simulink model "ROPOD_4Wheel_Tdistkinb_cntr_vel_filter_test"  (R2017b)
settings: Solver=FixedStepAuto  StartTime=0.0  StopTime=Inf  FixedStep=Ts  RelTol=1e-3
PreLoadFcn:
  | init_model
InitFcn:
  | init_model
values from neighbouring files (symbols this model uses):
  FFtheta_intia = 0    [init_model.m]
  FFxy_mass = 0*80    (= 0)    [init_model.m]
  max_hw_tau = 7.0    (= 7)    [init_model.m]
  max_ropod_sw_force = 500    [init_model.m]
  max_ropod_sw_tau = 250    [init_model.m]
  Nwheels = 4    [Jqwl_numeric_function.m]    (also in S_matrix.m; extract_kinmodel_parameters.m; init_model.m; tau_optimal_dist_vec_fun.m)
  pivot_offs_sws = [3.835 3.465 2.059 0.357]    [init_model.m]
  SW_COM1_ENABLE1 = hex2dec('0001')    [init_model.m]
  SW_COM1_ENABLE2 = hex2dec('0002')    [init_model.m]
  SW_COM1_MODE_TORQUE = bitshift(hex2dec('0000'),2)    [init_model.m]
  SW_COM1_MODE_VELOCITY = bitshift(hex2dec('0002'),2)    [init_model.m]
  SW_COM1_USE_TS = hex2dec('8000')    [init_model.m]
  sw_tau_2_curr = 1/motor_physical_parameters.torqueconstant.value    [init_model.m]
  Taucompfactor = 2.0    (= 2)    [init_model.m]
  Tinit = 5    [init_model.m]
  Ts = 0.001    [init_model.m]
  Tsp = 1    [init_model.m]
undefined symbols (not defined in the file or in its folder): DiscIntNeverNeededParam, Pose, ropod_kinmodel_param, Twist
libraries: robotlib x48, simulink x46, cstblocks x23, dspsigops x12, SOEM_EtherCAT_Lib x5, robotcorelib x1
(part 4 of 4)

== system ROPOD_4Wheel_Tdistkinb_cntr_vel_filter_test/Non-ROS Ropod Controller/wheel vel cntr/Wheels Velocity controller/G_I_LL_LPF Controller3/Shapeit Lead-Lag (Tustin) ==
  In : Inport
  fz : Inport  Port=2
  fp : Inport  Port=3
  Add : Sum  Inputs=+-
  Constant1 : Constant
  Constant2 : Constant  Value=0
  Constant4 : Constant
  Divide : Product  Inputs=*/
  Divide1 : Product  Inputs=/*
  Gain1 : Gain  Gain=2*pi
  Gain2 : Gain  Gain=2*pi
  PID Controller3 : simulink/Continuous/PID Controller  Controller=PID  TimeDomain=Discrete-time  SampleTime=Ts  IntegratorMethod=Trapezoidal  FilterMethod=Trapezoidal  Form=Parallel  UseFilter=on  ControllerParametersSource=external  P=0.4  I=0.4*2*pi*3  D=0  N=100  InitialConditionSource=internal  InitialConditionForIntegrator=0  InitialConditionForFilter=0  ExternalReset=none  LimitOutput=off  UpperSaturationLimit=max_hw_tau  LowerSaturationLimit=-max_hw_tau  LinearizeAsGain=on  AntiWindupMode=clamping  Kb=1  TrackingMode=off  Kt=1  PParamMin=[]  PParamMax=[]  IParamMin=[]  IParamMax=[]  DParamMin=[]  DParamMax=[]  NParamMin=[]  NParamMax=[]  KbParamMin=[]  KbParamMax=[]  KtParamMin=[]  KtParamMax=[]  POutMin=[]  POutMax=[]  IOutMin=[]  IOutMax=[]  DOutMin=[]  DOutMax=[]  NOutMin=[]  NOutMax=[]  KbOutMin=[]  KbOutMax=[]  KtOutMin=[]  KtOutMax=[]  IntegratorOutMin=[]  IntegratorOutMax=[]  FilterOutMin=[]  FilterOutMax=[]  SumOutMin=[]  SumOutMax=[]  SumI1OutMin=[]  SumI1OutMax=[]  SumI2OutMin=[]  SumI2OutMax=[]  SumI3OutMin=[]  SumI3OutMax=[]  SumDOutMin=[]  SumDOutMax=[]  SaturationOutMin=[]  SaturationOutMax=[]  IntegratorContinuousStateAttributes=''  IntegratorStateMustResolveToSignalObject=off  IntegratorRTWStateStorageClass=Auto  FilterContinuousStateAttributes=''  FilterStateMustResolveToSignalObject=off  FilterRTWStateStorageClass=Auto  DifferentiatorICPrevScaledInput=0  DifferentiatorOutMin=[]  DifferentiatorOutMax=[]  InitialConditionSetting=State (most efficient)  FilterDiffOutCoefMin=[]  FilterDiffOutCoefMax=[]  SumDenOutMin=[]  SumDenOutMax=[]  SumNumOutMin=[]  SumNumOutMax=[]  ReciprocalOutMin=[]  ReciprocalOutMax=[]  DivideOutMin=[]  DivideOutMax=[]  TunerSelectOption=Transfer Function Based (PID Tuner App)
  Out : Outport
  wires:
  Divide1/1 -> PID Controller3/4
  Add/1 -> Divide1/2
  Constant1/1 -> Add/1
  Divide/1 -> Add/2
  Gain2/1 -> Divide/1, Divide1/1
  Constant2/1 -> PID Controller3/3
  Gain1/1 -> Divide/2, PID Controller3/5
  fp/1 -> Gain1/1
  fz/1 -> Gain2/1
  PID Controller3/1 -> Out/1
  In/1 -> PID Controller3/1
  Constant4/1 -> PID Controller3/2

== system ROPOD_4Wheel_Tdistkinb_cntr_vel_filter_test/Non-ROS Ropod Controller/wheel vel cntr/Wheels Velocity controller/G_I_LL_LPF Controller4/Shapeit Integrator (Tustin) ==
  In : Inport
  I_fhz : Inport  Port=2
  reset : Inport  Port=3
  Constant : Constant  Value=0
  Constant4 : Constant
  Constant5 : Constant  Value=0
  Gain2 : Gain  Gain=2*pi
  PID Controller3 : simulink/Continuous/PID Controller  Controller=PID  TimeDomain=Discrete-time  SampleTime=Ts  IntegratorMethod=Trapezoidal  FilterMethod=Trapezoidal  Form=Parallel  UseFilter=on  ControllerParametersSource=external  P=0.4  I=0.4*2*pi*3  D=0  N=100  InitialConditionSource=internal  InitialConditionForIntegrator=0  InitialConditionForFilter=0  ExternalReset=level  LimitOutput=on  UpperSaturationLimit=max_hw_tau  LowerSaturationLimit=-max_hw_tau  LinearizeAsGain=on  AntiWindupMode=clamping  Kb=1  TrackingMode=off  Kt=1  PParamMin=[]  PParamMax=[]  IParamMin=[]  IParamMax=[]  DParamMin=[]  DParamMax=[]  NParamMin=[]  NParamMax=[]  KbParamMin=[]  KbParamMax=[]  KtParamMin=[]  KtParamMax=[]  POutMin=[]  POutMax=[]  IOutMin=[]  IOutMax=[]  DOutMin=[]  DOutMax=[]  NOutMin=[]  NOutMax=[]  KbOutMin=[]  KbOutMax=[]  KtOutMin=[]  KtOutMax=[]  IntegratorOutMin=[]  IntegratorOutMax=[]  FilterOutMin=[]  FilterOutMax=[]  SumOutMin=[]  SumOutMax=[]  SumI1OutMin=[]  SumI1OutMax=[]  SumI2OutMin=[]  SumI2OutMax=[]  SumI3OutMin=[]  SumI3OutMax=[]  SumDOutMin=[]  SumDOutMax=[]  SaturationOutMin=[]  SaturationOutMax=[]  IntegratorContinuousStateAttributes=''  IntegratorStateMustResolveToSignalObject=off  IntegratorRTWStateStorageClass=Auto  FilterContinuousStateAttributes=''  FilterStateMustResolveToSignalObject=off  FilterRTWStateStorageClass=Auto  DifferentiatorICPrevScaledInput=0  DifferentiatorOutMin=[]  DifferentiatorOutMax=[]  InitialConditionSetting=State (most efficient)  FilterDiffOutCoefMin=[]  FilterDiffOutCoefMax=[]  SumDenOutMin=[]  SumDenOutMax=[]  SumNumOutMin=[]  SumNumOutMax=[]  ReciprocalOutMin=[]  ReciprocalOutMax=[]  DivideOutMin=[]  DivideOutMax=[]  TunerSelectOption=Transfer Function Based (PID Tuner App)
  Product4 : Product
  Out : Outport
  wires:
  I_fhz/1 -> Product4/2
  Product4/1 -> Gain2/1
  reset/1 -> PID Controller3/6
  Gain2/1 -> PID Controller3/3
  PID Controller3/1 -> Out/1
  In/1 -> PID Controller3/1
  Constant4/1 -> Product4/1, PID Controller3/2
  Constant5/1 -> PID Controller3/5
  Constant/1 -> PID Controller3/4

== system ROPOD_4Wheel_Tdistkinb_cntr_vel_filter_test/Non-ROS Ropod Controller/wheel vel cntr/Wheels Velocity controller/G_I_LL_LPF Controller4/Shapeit Lead-Lag (Tustin) ==
  In : Inport
  fz : Inport  Port=2
  fp : Inport  Port=3
  Add : Sum  Inputs=+-
  Constant1 : Constant
  Constant2 : Constant  Value=0
  Constant4 : Constant
  Divide : Product  Inputs=*/
  Divide1 : Product  Inputs=/*
  Gain1 : Gain  Gain=2*pi
  Gain2 : Gain  Gain=2*pi
  PID Controller3 : simulink/Continuous/PID Controller  Controller=PID  TimeDomain=Discrete-time  SampleTime=Ts  IntegratorMethod=Trapezoidal  FilterMethod=Trapezoidal  Form=Parallel  UseFilter=on  ControllerParametersSource=external  P=0.4  I=0.4*2*pi*3  D=0  N=100  InitialConditionSource=internal  InitialConditionForIntegrator=0  InitialConditionForFilter=0  ExternalReset=none  LimitOutput=off  UpperSaturationLimit=max_hw_tau  LowerSaturationLimit=-max_hw_tau  LinearizeAsGain=on  AntiWindupMode=clamping  Kb=1  TrackingMode=off  Kt=1  PParamMin=[]  PParamMax=[]  IParamMin=[]  IParamMax=[]  DParamMin=[]  DParamMax=[]  NParamMin=[]  NParamMax=[]  KbParamMin=[]  KbParamMax=[]  KtParamMin=[]  KtParamMax=[]  POutMin=[]  POutMax=[]  IOutMin=[]  IOutMax=[]  DOutMin=[]  DOutMax=[]  NOutMin=[]  NOutMax=[]  KbOutMin=[]  KbOutMax=[]  KtOutMin=[]  KtOutMax=[]  IntegratorOutMin=[]  IntegratorOutMax=[]  FilterOutMin=[]  FilterOutMax=[]  SumOutMin=[]  SumOutMax=[]  SumI1OutMin=[]  SumI1OutMax=[]  SumI2OutMin=[]  SumI2OutMax=[]  SumI3OutMin=[]  SumI3OutMax=[]  SumDOutMin=[]  SumDOutMax=[]  SaturationOutMin=[]  SaturationOutMax=[]  IntegratorContinuousStateAttributes=''  IntegratorStateMustResolveToSignalObject=off  IntegratorRTWStateStorageClass=Auto  FilterContinuousStateAttributes=''  FilterStateMustResolveToSignalObject=off  FilterRTWStateStorageClass=Auto  DifferentiatorICPrevScaledInput=0  DifferentiatorOutMin=[]  DifferentiatorOutMax=[]  InitialConditionSetting=State (most efficient)  FilterDiffOutCoefMin=[]  FilterDiffOutCoefMax=[]  SumDenOutMin=[]  SumDenOutMax=[]  SumNumOutMin=[]  SumNumOutMax=[]  ReciprocalOutMin=[]  ReciprocalOutMax=[]  DivideOutMin=[]  DivideOutMax=[]  TunerSelectOption=Transfer Function Based (PID Tuner App)
  Out : Outport
  wires:
  Constant4/1 -> PID Controller3/2
  In/1 -> PID Controller3/1
  PID Controller3/1 -> Out/1
  fz/1 -> Gain2/1
  fp/1 -> Gain1/1
  Gain1/1 -> PID Controller3/5, Divide/2
  Constant2/1 -> PID Controller3/3
  Gain2/1 -> Divide1/1, Divide/1
  Divide/1 -> Add/2
  Constant1/1 -> Add/1
  Add/1 -> Divide1/2
  Divide1/1 -> PID Controller3/4

== system ROPOD_4Wheel_Tdistkinb_cntr_vel_filter_test/Non-ROS Ropod Controller/wheel vel cntr/Wheels Velocity controller/G_I_LL_LPF Controller5/Shapeit Integrator (Tustin) ==
  In : Inport
  I_fhz : Inport  Port=2
  reset : Inport  Port=3
  Constant : Constant  Value=0
  Constant4 : Constant
  Constant5 : Constant  Value=0
  Gain2 : Gain  Gain=2*pi
  PID Controller3 : simulink/Continuous/PID Controller  Controller=PID  TimeDomain=Discrete-time  SampleTime=Ts  IntegratorMethod=Trapezoidal  FilterMethod=Trapezoidal  Form=Parallel  UseFilter=on  ControllerParametersSource=external  P=0.4  I=0.4*2*pi*3  D=0  N=100  InitialConditionSource=internal  InitialConditionForIntegrator=0  InitialConditionForFilter=0  ExternalReset=level  LimitOutput=on  UpperSaturationLimit=max_hw_tau  LowerSaturationLimit=-max_hw_tau  LinearizeAsGain=on  AntiWindupMode=clamping  Kb=1  TrackingMode=off  Kt=1  PParamMin=[]  PParamMax=[]  IParamMin=[]  IParamMax=[]  DParamMin=[]  DParamMax=[]  NParamMin=[]  NParamMax=[]  KbParamMin=[]  KbParamMax=[]  KtParamMin=[]  KtParamMax=[]  POutMin=[]  POutMax=[]  IOutMin=[]  IOutMax=[]  DOutMin=[]  DOutMax=[]  NOutMin=[]  NOutMax=[]  KbOutMin=[]  KbOutMax=[]  KtOutMin=[]  KtOutMax=[]  IntegratorOutMin=[]  IntegratorOutMax=[]  FilterOutMin=[]  FilterOutMax=[]  SumOutMin=[]  SumOutMax=[]  SumI1OutMin=[]  SumI1OutMax=[]  SumI2OutMin=[]  SumI2OutMax=[]  SumI3OutMin=[]  SumI3OutMax=[]  SumDOutMin=[]  SumDOutMax=[]  SaturationOutMin=[]  SaturationOutMax=[]  IntegratorContinuousStateAttributes=''  IntegratorStateMustResolveToSignalObject=off  IntegratorRTWStateStorageClass=Auto  FilterContinuousStateAttributes=''  FilterStateMustResolveToSignalObject=off  FilterRTWStateStorageClass=Auto  DifferentiatorICPrevScaledInput=0  DifferentiatorOutMin=[]  DifferentiatorOutMax=[]  InitialConditionSetting=State (most efficient)  FilterDiffOutCoefMin=[]  FilterDiffOutCoefMax=[]  SumDenOutMin=[]  SumDenOutMax=[]  SumNumOutMin=[]  SumNumOutMax=[]  ReciprocalOutMin=[]  ReciprocalOutMax=[]  DivideOutMin=[]  DivideOutMax=[]  TunerSelectOption=Transfer Function Based (PID Tuner App)
  Product4 : Product
  Out : Outport
  wires:
  Constant/1 -> PID Controller3/4
  Constant5/1 -> PID Controller3/5
  Constant4/1 -> PID Controller3/2, Product4/1
  In/1 -> PID Controller3/1
  PID Controller3/1 -> Out/1
  Gain2/1 -> PID Controller3/3
  reset/1 -> PID Controller3/6
  Product4/1 -> Gain2/1
  I_fhz/1 -> Product4/2

== system ROPOD_4Wheel_Tdistkinb_cntr_vel_filter_test/Non-ROS Ropod Controller/wheel vel cntr/Wheels Velocity controller/G_I_LL_LPF Controller5/Shapeit Lead-Lag (Tustin) ==
  In : Inport
  fz : Inport  Port=2
  fp : Inport  Port=3
  Add : Sum  Inputs=+-
  Constant1 : Constant
  Constant2 : Constant  Value=0
  Constant4 : Constant
  Divide : Product  Inputs=*/
  Divide1 : Product  Inputs=/*
  Gain1 : Gain  Gain=2*pi
  Gain2 : Gain  Gain=2*pi
  PID Controller3 : simulink/Continuous/PID Controller  Controller=PID  TimeDomain=Discrete-time  SampleTime=Ts  IntegratorMethod=Trapezoidal  FilterMethod=Trapezoidal  Form=Parallel  UseFilter=on  ControllerParametersSource=external  P=0.4  I=0.4*2*pi*3  D=0  N=100  InitialConditionSource=internal  InitialConditionForIntegrator=0  InitialConditionForFilter=0  ExternalReset=none  LimitOutput=off  UpperSaturationLimit=max_hw_tau  LowerSaturationLimit=-max_hw_tau  LinearizeAsGain=on  AntiWindupMode=clamping  Kb=1  TrackingMode=off  Kt=1  PParamMin=[]  PParamMax=[]  IParamMin=[]  IParamMax=[]  DParamMin=[]  DParamMax=[]  NParamMin=[]  NParamMax=[]  KbParamMin=[]  KbParamMax=[]  KtParamMin=[]  KtParamMax=[]  POutMin=[]  POutMax=[]  IOutMin=[]  IOutMax=[]  DOutMin=[]  DOutMax=[]  NOutMin=[]  NOutMax=[]  KbOutMin=[]  KbOutMax=[]  KtOutMin=[]  KtOutMax=[]  IntegratorOutMin=[]  IntegratorOutMax=[]  FilterOutMin=[]  FilterOutMax=[]  SumOutMin=[]  SumOutMax=[]  SumI1OutMin=[]  SumI1OutMax=[]  SumI2OutMin=[]  SumI2OutMax=[]  SumI3OutMin=[]  SumI3OutMax=[]  SumDOutMin=[]  SumDOutMax=[]  SaturationOutMin=[]  SaturationOutMax=[]  IntegratorContinuousStateAttributes=''  IntegratorStateMustResolveToSignalObject=off  IntegratorRTWStateStorageClass=Auto  FilterContinuousStateAttributes=''  FilterStateMustResolveToSignalObject=off  FilterRTWStateStorageClass=Auto  DifferentiatorICPrevScaledInput=0  DifferentiatorOutMin=[]  DifferentiatorOutMax=[]  InitialConditionSetting=State (most efficient)  FilterDiffOutCoefMin=[]  FilterDiffOutCoefMax=[]  SumDenOutMin=[]  SumDenOutMax=[]  SumNumOutMin=[]  SumNumOutMax=[]  ReciprocalOutMin=[]  ReciprocalOutMax=[]  DivideOutMin=[]  DivideOutMax=[]  TunerSelectOption=Transfer Function Based (PID Tuner App)
  Out : Outport
  wires:
  Divide1/1 -> PID Controller3/4
  Add/1 -> Divide1/2
  Constant1/1 -> Add/1
  Divide/1 -> Add/2
  Gain2/1 -> Divide/1, Divide1/1
  Constant2/1 -> PID Controller3/3
  Gain1/1 -> Divide/2, PID Controller3/5
  fp/1 -> Gain1/1
  fz/1 -> Gain2/1
  PID Controller3/1 -> Out/1
  In/1 -> PID Controller3/1
  Constant4/1 -> PID Controller3/2

== system ROPOD_4Wheel_Tdistkinb_cntr_vel_filter_test/Non-ROS Ropod Controller/wheel vel cntr/Wheels Velocity controller/G_I_LL_LPF Controller6/Shapeit Integrator (Tustin) ==
  In : Inport
  I_fhz : Inport  Port=2
  reset : Inport  Port=3
  Constant : Constant  Value=0
  Constant4 : Constant
  Constant5 : Constant  Value=0
  Gain2 : Gain  Gain=2*pi
  PID Controller3 : simulink/Continuous/PID Controller  Controller=PID  TimeDomain=Discrete-time  SampleTime=Ts  IntegratorMethod=Trapezoidal  FilterMethod=Trapezoidal  Form=Parallel  UseFilter=on  ControllerParametersSource=external  P=0.4  I=0.4*2*pi*3  D=0  N=100  InitialConditionSource=internal  InitialConditionForIntegrator=0  InitialConditionForFilter=0  ExternalReset=level  LimitOutput=on  UpperSaturationLimit=max_hw_tau  LowerSaturationLimit=-max_hw_tau  LinearizeAsGain=on  AntiWindupMode=clamping  Kb=1  TrackingMode=off  Kt=1  PParamMin=[]  PParamMax=[]  IParamMin=[]  IParamMax=[]  DParamMin=[]  DParamMax=[]  NParamMin=[]  NParamMax=[]  KbParamMin=[]  KbParamMax=[]  KtParamMin=[]  KtParamMax=[]  POutMin=[]  POutMax=[]  IOutMin=[]  IOutMax=[]  DOutMin=[]  DOutMax=[]  NOutMin=[]  NOutMax=[]  KbOutMin=[]  KbOutMax=[]  KtOutMin=[]  KtOutMax=[]  IntegratorOutMin=[]  IntegratorOutMax=[]  FilterOutMin=[]  FilterOutMax=[]  SumOutMin=[]  SumOutMax=[]  SumI1OutMin=[]  SumI1OutMax=[]  SumI2OutMin=[]  SumI2OutMax=[]  SumI3OutMin=[]  SumI3OutMax=[]  SumDOutMin=[]  SumDOutMax=[]  SaturationOutMin=[]  SaturationOutMax=[]  IntegratorContinuousStateAttributes=''  IntegratorStateMustResolveToSignalObject=off  IntegratorRTWStateStorageClass=Auto  FilterContinuousStateAttributes=''  FilterStateMustResolveToSignalObject=off  FilterRTWStateStorageClass=Auto  DifferentiatorICPrevScaledInput=0  DifferentiatorOutMin=[]  DifferentiatorOutMax=[]  InitialConditionSetting=State (most efficient)  FilterDiffOutCoefMin=[]  FilterDiffOutCoefMax=[]  SumDenOutMin=[]  SumDenOutMax=[]  SumNumOutMin=[]  SumNumOutMax=[]  ReciprocalOutMin=[]  ReciprocalOutMax=[]  DivideOutMin=[]  DivideOutMax=[]  TunerSelectOption=Transfer Function Based (PID Tuner App)
  Product4 : Product
  Out : Outport
  wires:
  I_fhz/1 -> Product4/2
  Product4/1 -> Gain2/1
  reset/1 -> PID Controller3/6
  Gain2/1 -> PID Controller3/3
  PID Controller3/1 -> Out/1
  In/1 -> PID Controller3/1
  Constant4/1 -> Product4/1, PID Controller3/2
  Constant5/1 -> PID Controller3/5
  Constant/1 -> PID Controller3/4

== system ROPOD_4Wheel_Tdistkinb_cntr_vel_filter_test/Non-ROS Ropod Controller/wheel vel cntr/Wheels Velocity controller/G_I_LL_LPF Controller6/Shapeit Lead-Lag (Tustin) ==
  In : Inport
  fz : Inport  Port=2
  fp : Inport  Port=3
  Add : Sum  Inputs=+-
  Constant1 : Constant
  Constant2 : Constant  Value=0
  Constant4 : Constant
  Divide : Product  Inputs=*/
  Divide1 : Product  Inputs=/*
  Gain1 : Gain  Gain=2*pi
  Gain2 : Gain  Gain=2*pi
  PID Controller3 : simulink/Continuous/PID Controller  Controller=PID  TimeDomain=Discrete-time  SampleTime=Ts  IntegratorMethod=Trapezoidal  FilterMethod=Trapezoidal  Form=Parallel  UseFilter=on  ControllerParametersSource=external  P=0.4  I=0.4*2*pi*3  D=0  N=100  InitialConditionSource=internal  InitialConditionForIntegrator=0  InitialConditionForFilter=0  ExternalReset=none  LimitOutput=off  UpperSaturationLimit=max_hw_tau  LowerSaturationLimit=-max_hw_tau  LinearizeAsGain=on  AntiWindupMode=clamping  Kb=1  TrackingMode=off  Kt=1  PParamMin=[]  PParamMax=[]  IParamMin=[]  IParamMax=[]  DParamMin=[]  DParamMax=[]  NParamMin=[]  NParamMax=[]  KbParamMin=[]  KbParamMax=[]  KtParamMin=[]  KtParamMax=[]  POutMin=[]  POutMax=[]  IOutMin=[]  IOutMax=[]  DOutMin=[]  DOutMax=[]  NOutMin=[]  NOutMax=[]  KbOutMin=[]  KbOutMax=[]  KtOutMin=[]  KtOutMax=[]  IntegratorOutMin=[]  IntegratorOutMax=[]  FilterOutMin=[]  FilterOutMax=[]  SumOutMin=[]  SumOutMax=[]  SumI1OutMin=[]  SumI1OutMax=[]  SumI2OutMin=[]  SumI2OutMax=[]  SumI3OutMin=[]  SumI3OutMax=[]  SumDOutMin=[]  SumDOutMax=[]  SaturationOutMin=[]  SaturationOutMax=[]  IntegratorContinuousStateAttributes=''  IntegratorStateMustResolveToSignalObject=off  IntegratorRTWStateStorageClass=Auto  FilterContinuousStateAttributes=''  FilterStateMustResolveToSignalObject=off  FilterRTWStateStorageClass=Auto  DifferentiatorICPrevScaledInput=0  DifferentiatorOutMin=[]  DifferentiatorOutMax=[]  InitialConditionSetting=State (most efficient)  FilterDiffOutCoefMin=[]  FilterDiffOutCoefMax=[]  SumDenOutMin=[]  SumDenOutMax=[]  SumNumOutMin=[]  SumNumOutMax=[]  ReciprocalOutMin=[]  ReciprocalOutMax=[]  DivideOutMin=[]  DivideOutMax=[]  TunerSelectOption=Transfer Function Based (PID Tuner App)
  Out : Outport
  wires:
  Constant4/1 -> PID Controller3/2
  In/1 -> PID Controller3/1
  PID Controller3/1 -> Out/1
  fz/1 -> Gain2/1
  fp/1 -> Gain1/1
  Gain1/1 -> PID Controller3/5, Divide/2
  Constant2/1 -> PID Controller3/3
  Gain2/1 -> Divide1/1, Divide/1
  Divide/1 -> Add/2
  Constant1/1 -> Add/1
  Add/1 -> Divide1/2
  Divide1/1 -> PID Controller3/4

== system ROPOD_4Wheel_Tdistkinb_cntr_vel_filter_test/Non-ROS Ropod Controller/wheel vel cntr/Wheels Velocity controller/G_I_LL_LPF Controller7/Shapeit Integrator (Tustin) ==
  In : Inport
  I_fhz : Inport  Port=2
  reset : Inport  Port=3
  Constant : Constant  Value=0
  Constant4 : Constant
  Constant5 : Constant  Value=0
  Gain2 : Gain  Gain=2*pi
  PID Controller3 : simulink/Continuous/PID Controller  Controller=PID  TimeDomain=Discrete-time  SampleTime=Ts  IntegratorMethod=Trapezoidal  FilterMethod=Trapezoidal  Form=Parallel  UseFilter=on  ControllerParametersSource=external  P=0.4  I=0.4*2*pi*3  D=0  N=100  InitialConditionSource=internal  InitialConditionForIntegrator=0  InitialConditionForFilter=0  ExternalReset=level  LimitOutput=on  UpperSaturationLimit=max_hw_tau  LowerSaturationLimit=-max_hw_tau  LinearizeAsGain=on  AntiWindupMode=clamping  Kb=1  TrackingMode=off  Kt=1  PParamMin=[]  PParamMax=[]  IParamMin=[]  IParamMax=[]  DParamMin=[]  DParamMax=[]  NParamMin=[]  NParamMax=[]  KbParamMin=[]  KbParamMax=[]  KtParamMin=[]  KtParamMax=[]  POutMin=[]  POutMax=[]  IOutMin=[]  IOutMax=[]  DOutMin=[]  DOutMax=[]  NOutMin=[]  NOutMax=[]  KbOutMin=[]  KbOutMax=[]  KtOutMin=[]  KtOutMax=[]  IntegratorOutMin=[]  IntegratorOutMax=[]  FilterOutMin=[]  FilterOutMax=[]  SumOutMin=[]  SumOutMax=[]  SumI1OutMin=[]  SumI1OutMax=[]  SumI2OutMin=[]  SumI2OutMax=[]  SumI3OutMin=[]  SumI3OutMax=[]  SumDOutMin=[]  SumDOutMax=[]  SaturationOutMin=[]  SaturationOutMax=[]  IntegratorContinuousStateAttributes=''  IntegratorStateMustResolveToSignalObject=off  IntegratorRTWStateStorageClass=Auto  FilterContinuousStateAttributes=''  FilterStateMustResolveToSignalObject=off  FilterRTWStateStorageClass=Auto  DifferentiatorICPrevScaledInput=0  DifferentiatorOutMin=[]  DifferentiatorOutMax=[]  InitialConditionSetting=State (most efficient)  FilterDiffOutCoefMin=[]  FilterDiffOutCoefMax=[]  SumDenOutMin=[]  SumDenOutMax=[]  SumNumOutMin=[]  SumNumOutMax=[]  ReciprocalOutMin=[]  ReciprocalOutMax=[]  DivideOutMin=[]  DivideOutMax=[]  TunerSelectOption=Transfer Function Based (PID Tuner App)
  Product4 : Product
  Out : Outport
  wires:
  Constant/1 -> PID Controller3/4
  Constant5/1 -> PID Controller3/5
  Constant4/1 -> PID Controller3/2, Product4/1
  In/1 -> PID Controller3/1
  PID Controller3/1 -> Out/1
  Gain2/1 -> PID Controller3/3
  reset/1 -> PID Controller3/6
  Product4/1 -> Gain2/1
  I_fhz/1 -> Product4/2

== system ROPOD_4Wheel_Tdistkinb_cntr_vel_filter_test/Non-ROS Ropod Controller/wheel vel cntr/Wheels Velocity controller/G_I_LL_LPF Controller7/Shapeit Lead-Lag (Tustin) ==
  In : Inport
  fz : Inport  Port=2
  fp : Inport  Port=3
  Add : Sum  Inputs=+-
  Constant1 : Constant
  Constant2 : Constant  Value=0
  Constant4 : Constant
  Divide : Product  Inputs=*/
  Divide1 : Product  Inputs=/*
  Gain1 : Gain  Gain=2*pi
  Gain2 : Gain  Gain=2*pi
  PID Controller3 : simulink/Continuous/PID Controller  Controller=PID  TimeDomain=Discrete-time  SampleTime=Ts  IntegratorMethod=Trapezoidal  FilterMethod=Trapezoidal  Form=Parallel  UseFilter=on  ControllerParametersSource=external  P=0.4  I=0.4*2*pi*3  D=0  N=100  InitialConditionSource=internal  InitialConditionForIntegrator=0  InitialConditionForFilter=0  ExternalReset=none  LimitOutput=off  UpperSaturationLimit=max_hw_tau  LowerSaturationLimit=-max_hw_tau  LinearizeAsGain=on  AntiWindupMode=clamping  Kb=1  TrackingMode=off  Kt=1  PParamMin=[]  PParamMax=[]  IParamMin=[]  IParamMax=[]  DParamMin=[]  DParamMax=[]  NParamMin=[]  NParamMax=[]  KbParamMin=[]  KbParamMax=[]  KtParamMin=[]  KtParamMax=[]  POutMin=[]  POutMax=[]  IOutMin=[]  IOutMax=[]  DOutMin=[]  DOutMax=[]  NOutMin=[]  NOutMax=[]  KbOutMin=[]  KbOutMax=[]  KtOutMin=[]  KtOutMax=[]  IntegratorOutMin=[]  IntegratorOutMax=[]  FilterOutMin=[]  FilterOutMax=[]  SumOutMin=[]  SumOutMax=[]  SumI1OutMin=[]  SumI1OutMax=[]  SumI2OutMin=[]  SumI2OutMax=[]  SumI3OutMin=[]  SumI3OutMax=[]  SumDOutMin=[]  SumDOutMax=[]  SaturationOutMin=[]  SaturationOutMax=[]  IntegratorContinuousStateAttributes=''  IntegratorStateMustResolveToSignalObject=off  IntegratorRTWStateStorageClass=Auto  FilterContinuousStateAttributes=''  FilterStateMustResolveToSignalObject=off  FilterRTWStateStorageClass=Auto  DifferentiatorICPrevScaledInput=0  DifferentiatorOutMin=[]  DifferentiatorOutMax=[]  InitialConditionSetting=State (most efficient)  FilterDiffOutCoefMin=[]  FilterDiffOutCoefMax=[]  SumDenOutMin=[]  SumDenOutMax=[]  SumNumOutMin=[]  SumNumOutMax=[]  ReciprocalOutMin=[]  ReciprocalOutMax=[]  DivideOutMin=[]  DivideOutMax=[]  TunerSelectOption=Transfer Function Based (PID Tuner App)
  Out : Outport
  wires:
  Divide1/1 -> PID Controller3/4
  Add/1 -> Divide1/2
  Constant1/1 -> Add/1
  Divide/1 -> Add/2
  Gain2/1 -> Divide/1, Divide1/1
  Constant2/1 -> PID Controller3/3
  Gain1/1 -> Divide/2, PID Controller3/5
  fp/1 -> Gain1/1
  fz/1 -> Gain2/1
  PID Controller3/1 -> Out/1
  In/1 -> PID Controller3/1
  Constant4/1 -> PID Controller3/2

== system ROPOD_4Wheel_Tdistkinb_cntr_vel_filter_test/Non-ROS Ropod Controller/wheel vel cntr/Wheels Velocity controller/G_I_LL_LPF Controller8/Shapeit Integrator (Tustin) ==
  In : Inport
  I_fhz : Inport  Port=2
  reset : Inport  Port=3
  Constant : Constant  Value=0
  Constant4 : Constant
  Constant5 : Constant  Value=0
  Gain2 : Gain  Gain=2*pi
  PID Controller3 : simulink/Continuous/PID Controller  Controller=PID  TimeDomain=Discrete-time  SampleTime=Ts  IntegratorMethod=Trapezoidal  FilterMethod=Trapezoidal  Form=Parallel  UseFilter=on  ControllerParametersSource=external  P=0.4  I=0.4*2*pi*3  D=0  N=100  InitialConditionSource=internal  InitialConditionForIntegrator=0  InitialConditionForFilter=0  ExternalReset=level  LimitOutput=on  UpperSaturationLimit=max_hw_tau  LowerSaturationLimit=-max_hw_tau  LinearizeAsGain=on  AntiWindupMode=clamping  Kb=1  TrackingMode=off  Kt=1  PParamMin=[]  PParamMax=[]  IParamMin=[]  IParamMax=[]  DParamMin=[]  DParamMax=[]  NParamMin=[]  NParamMax=[]  KbParamMin=[]  KbParamMax=[]  KtParamMin=[]  KtParamMax=[]  POutMin=[]  POutMax=[]  IOutMin=[]  IOutMax=[]  DOutMin=[]  DOutMax=[]  NOutMin=[]  NOutMax=[]  KbOutMin=[]  KbOutMax=[]  KtOutMin=[]  KtOutMax=[]  IntegratorOutMin=[]  IntegratorOutMax=[]  FilterOutMin=[]  FilterOutMax=[]  SumOutMin=[]  SumOutMax=[]  SumI1OutMin=[]  SumI1OutMax=[]  SumI2OutMin=[]  SumI2OutMax=[]  SumI3OutMin=[]  SumI3OutMax=[]  SumDOutMin=[]  SumDOutMax=[]  SaturationOutMin=[]  SaturationOutMax=[]  IntegratorContinuousStateAttributes=''  IntegratorStateMustResolveToSignalObject=off  IntegratorRTWStateStorageClass=Auto  FilterContinuousStateAttributes=''  FilterStateMustResolveToSignalObject=off  FilterRTWStateStorageClass=Auto  DifferentiatorICPrevScaledInput=0  DifferentiatorOutMin=[]  DifferentiatorOutMax=[]  InitialConditionSetting=State (most efficient)  FilterDiffOutCoefMin=[]  FilterDiffOutCoefMax=[]  SumDenOutMin=[]  SumDenOutMax=[]  SumNumOutMin=[]  SumNumOutMax=[]  ReciprocalOutMin=[]  ReciprocalOutMax=[]  DivideOutMin=[]  DivideOutMax=[]  TunerSelectOption=Transfer Function Based (PID Tuner App)
  Product4 : Product
  Out : Outport
  wires:
  I_fhz/1 -> Product4/2
  Product4/1 -> Gain2/1
  reset/1 -> PID Controller3/6
  Gain2/1 -> PID Controller3/3
  PID Controller3/1 -> Out/1
  In/1 -> PID Controller3/1
  Constant4/1 -> Product4/1, PID Controller3/2
  Constant5/1 -> PID Controller3/5
  Constant/1 -> PID Controller3/4

== system ROPOD_4Wheel_Tdistkinb_cntr_vel_filter_test/Non-ROS Ropod Controller/wheel vel cntr/Wheels Velocity controller/G_I_LL_LPF Controller8/Shapeit Lead-Lag (Tustin) ==
  In : Inport
  fz : Inport  Port=2
  fp : Inport  Port=3
  Add : Sum  Inputs=+-
  Constant1 : Constant
  Constant2 : Constant  Value=0
  Constant4 : Constant
  Divide : Product  Inputs=*/
  Divide1 : Product  Inputs=/*
  Gain1 : Gain  Gain=2*pi
  Gain2 : Gain  Gain=2*pi
  PID Controller3 : simulink/Continuous/PID Controller  Controller=PID  TimeDomain=Discrete-time  SampleTime=Ts  IntegratorMethod=Trapezoidal  FilterMethod=Trapezoidal  Form=Parallel  UseFilter=on  ControllerParametersSource=external  P=0.4  I=0.4*2*pi*3  D=0  N=100  InitialConditionSource=internal  InitialConditionForIntegrator=0  InitialConditionForFilter=0  ExternalReset=none  LimitOutput=off  UpperSaturationLimit=max_hw_tau  LowerSaturationLimit=-max_hw_tau  LinearizeAsGain=on  AntiWindupMode=clamping  Kb=1  TrackingMode=off  Kt=1  PParamMin=[]  PParamMax=[]  IParamMin=[]  IParamMax=[]  DParamMin=[]  DParamMax=[]  NParamMin=[]  NParamMax=[]  KbParamMin=[]  KbParamMax=[]  KtParamMin=[]  KtParamMax=[]  POutMin=[]  POutMax=[]  IOutMin=[]  IOutMax=[]  DOutMin=[]  DOutMax=[]  NOutMin=[]  NOutMax=[]  KbOutMin=[]  KbOutMax=[]  KtOutMin=[]  KtOutMax=[]  IntegratorOutMin=[]  IntegratorOutMax=[]  FilterOutMin=[]  FilterOutMax=[]  SumOutMin=[]  SumOutMax=[]  SumI1OutMin=[]  SumI1OutMax=[]  SumI2OutMin=[]  SumI2OutMax=[]  SumI3OutMin=[]  SumI3OutMax=[]  SumDOutMin=[]  SumDOutMax=[]  SaturationOutMin=[]  SaturationOutMax=[]  IntegratorContinuousStateAttributes=''  IntegratorStateMustResolveToSignalObject=off  IntegratorRTWStateStorageClass=Auto  FilterContinuousStateAttributes=''  FilterStateMustResolveToSignalObject=off  FilterRTWStateStorageClass=Auto  DifferentiatorICPrevScaledInput=0  DifferentiatorOutMin=[]  DifferentiatorOutMax=[]  InitialConditionSetting=State (most efficient)  FilterDiffOutCoefMin=[]  FilterDiffOutCoefMax=[]  SumDenOutMin=[]  SumDenOutMax=[]  SumNumOutMin=[]  SumNumOutMax=[]  ReciprocalOutMin=[]  ReciprocalOutMax=[]  DivideOutMin=[]  DivideOutMax=[]  TunerSelectOption=Transfer Function Based (PID Tuner App)
  Out : Outport
  wires:
  Constant4/1 -> PID Controller3/2
  In/1 -> PID Controller3/1
  PID Controller3/1 -> Out/1
  fz/1 -> Gain2/1
  fp/1 -> Gain1/1
  Gain1/1 -> PID Controller3/5, Divide/2
  Constant2/1 -> PID Controller3/3
  Gain2/1 -> Divide1/1, Divide/1
  Divide/1 -> Add/2
  Constant1/1 -> Add/1
  Add/1 -> Divide1/2
  Divide1/1 -> PID Controller3/4

== matlab function ROPOD_4Wheel_Tdistkinb_cntr_vel_filter_test/Non-ROS Ropod Controller/ROPOD 4SW TORQUE_MODE/ROPOD_4Wheel_sens/Glitch removal + LP filter1/Remove_glitches1 ==
  data: vel input; Ts input; encoder input; encoder_out output
function encoder_out  = remove_glitches(vel, Ts, encoder)

persistent last_valid_encoder;
persistent invalid_cnt;

if(isempty(last_valid_encoder))
    last_valid_encoder = encoder;
    invalid_cnt = 0;
end

if abs( (last_valid_encoder-encoder)/Ts ) > 50 % maximum expected velocity rad/sec (2.5 m/s)
    encoder_out = last_valid_encoder + vel*Ts;    
    invalid_cnt = invalid_cnt +1;
else
    invalid_cnt = 0;
    encoder_out = encoder;
end

if invalid_cnt>1 
    invalid_cnt = 0;
    encoder_out = encoder;
end

last_valid_encoder = encoder_out;

== matlab function ROPOD_4Wheel_Tdistkinb_cntr_vel_filter_test/Non-ROS Ropod Controller/ROPOD 4SW TORQUE_MODE/ROPOD_4Wheel_sens/Glitch removal + LP filter/Remove_glitches1 ==
  data: vel input; Ts input; encoder input; encoder_out output
function encoder_out  = remove_glitches(vel, Ts, encoder)

persistent last_valid_encoder;
persistent invalid_cnt;

if(isempty(last_valid_encoder))
    last_valid_encoder = encoder;
    invalid_cnt = 0;
end

if abs( (last_valid_encoder-encoder)/Ts ) > 50 % maximum expected velocity rad/sec (2.5 m/s)
    encoder_out = last_valid_encoder + vel*Ts;    
    invalid_cnt = invalid_cnt +1;
else
    invalid_cnt = 0;
    encoder_out = encoder;
end

if invalid_cnt>1 
    invalid_cnt = 0;
    encoder_out = encoder;
end

last_valid_encoder = encoder_out;

== matlab function ROPOD_4Wheel_Tdistkinb_cntr_vel_filter_test/Non-ROS Ropod Controller/ROPOD 4SW TORQUE_MODE/ROPOD_4Wheel_sens/Glitch removal + LP filter2/Remove_glitches1 ==
  data: vel input; Ts input; encoder input; encoder_out output
function encoder_out  = remove_glitches(vel, Ts, encoder)

persistent last_valid_encoder;
persistent invalid_cnt;

if(isempty(last_valid_encoder))
    last_valid_encoder = encoder;
    invalid_cnt = 0;
end

if abs( (last_valid_encoder-encoder)/Ts ) > 50 % maximum expected velocity rad/sec (2.5 m/s)
    encoder_out = last_valid_encoder + vel*Ts;    
    invalid_cnt = invalid_cnt +1;
else
    invalid_cnt = 0;
    encoder_out = encoder;
end

if invalid_cnt>1 
    invalid_cnt = 0;
    encoder_out = encoder;
end

last_valid_encoder = encoder_out;

== matlab function ROPOD_4Wheel_Tdistkinb_cntr_vel_filter_test/Non-ROS Ropod Controller/ROPOD 4SW TORQUE_MODE/ROPOD_4Wheel_sens/Glitch removal + LP filter3/Remove_glitches1 ==
  data: vel input; Ts input; encoder input; encoder_out output
function encoder_out  = remove_glitches(vel, Ts, encoder)

persistent last_valid_encoder;
persistent invalid_cnt;

if(isempty(last_valid_encoder))
    last_valid_encoder = encoder;
    invalid_cnt = 0;
end

if abs( (last_valid_encoder-encoder)/Ts ) > 50 % maximum expected velocity rad/sec (2.5 m/s)
    encoder_out = last_valid_encoder + vel*Ts;    
    invalid_cnt = invalid_cnt +1;
else
    invalid_cnt = 0;
    encoder_out = encoder;
end

if invalid_cnt>1 
    invalid_cnt = 0;
    encoder_out = encoder;
end

last_valid_encoder = encoder_out;

== matlab function ROPOD_4Wheel_Tdistkinb_cntr_vel_filter_test/Non-ROS Ropod Controller/ROPOD 4SW TORQUE_MODE/ROPOD_4Wheel_sens/Glitch removal + LP filter4/Remove_glitches1 ==
  data: vel input; Ts input; encoder input; encoder_out output
function encoder_out  = remove_glitches(vel, Ts, encoder)

persistent last_valid_encoder;
persistent invalid_cnt;

if(isempty(last_valid_encoder))
    last_valid_encoder = encoder;
    invalid_cnt = 0;
end

if abs( (last_valid_encoder-encoder)/Ts ) > 50 % maximum expected velocity rad/sec (2.5 m/s)
    encoder_out = last_valid_encoder + vel*Ts;    
    invalid_cnt = invalid_cnt +1;
else
    invalid_cnt = 0;
    encoder_out = encoder;
end

if invalid_cnt>1 
    invalid_cnt = 0;
    encoder_out = encoder;
end

last_valid_encoder = encoder_out;

== matlab function ROPOD_4Wheel_Tdistkinb_cntr_vel_filter_test/Non-ROS Ropod Controller/Odometry and Measurement model 4SW/Jqwl_matrix ==
  data: ropod_kinmodel_param_vec input; Jqwl output; delta input
function Jqwl = Jqwl_matrix_wrapper(ropod_kinmodel_param_vec, delta)

Jqwl = Jqwl_matrix_wrapper(ropod_kinmodel_param_vec, delta);

end

== matlab function ROPOD_4Wheel_Tdistkinb_cntr_vel_filter_test/Non-ROS Ropod Controller/Odometry and Measurement model 4SW/pos_rot_matrix ==
  data: dqr_loc input; theta_odom input; dqr_glb output
function dqr_glb   = zrot(dqr_loc, theta_odom)
%ROPOD_JACOBIAN Summary of this function goes here
%   Detailed explanation goes here


dqr_glb = [  cos(theta_odom) -sin(theta_odom) 0; 
            sin(theta_odom)  cos(theta_odom) 0;
                    0             0  1]*dqr_loc;
end

== matlab function ROPOD_4Wheel_Tdistkinb_cntr_vel_filter_test/Non-ROS Ropod Controller/platform vel cntr/Inverse Kinematics 4SW/Gl_matrix ==
  data: ropod_kinmodel_param_vec input; Gl output; delta input
function Gl = Gl_matrix_wrapper(ropod_kinmodel_param_vec, delta)

Gl = Gl_matrix_wrapper(ropod_kinmodel_param_vec, delta);

end

== matlab function ROPOD_4Wheel_Tdistkinb_cntr_vel_filter_test/Non-ROS Ropod Controller/platform vel cntr/Torque distribution/Gl_matrices ==
  data: ropod_kinmodel_param_vec input; Gl output; delta input; Gtl output; GtSl output
function [Gl, Gtl, GtSl]   = G_matrices( ropod_kinmodel_param_vec, delta)
%ROPOD_JACOBIAN Summary of this function goes here
%   Detailed explanation goes here


Gl    = Gl_matrix_wrapper(ropod_kinmodel_param_vec, delta);
Gtl   = Gl.';
GtSl  = Gtl*S_matrix();
end

== matlab function ROPOD_4Wheel_Tdistkinb_cntr_vel_filter_test/Non-ROS Ropod Controller/ROPOD 4SW TORQUE_MODE/ROPOD_4Wheel_sens/Glitch removal + LP filter5/Remove_glitches1 ==
  data: vel input; Ts input; encoder input; encoder_out output
function encoder_out  = remove_glitches(vel, Ts, encoder)

persistent last_valid_encoder;
persistent invalid_cnt;

if(isempty(last_valid_encoder))
    last_valid_encoder = encoder;
    invalid_cnt = 0;
end

if abs( (last_valid_encoder-encoder)/Ts ) > 50 % maximum expected velocity rad/sec (2.5 m/s)
    encoder_out = last_valid_encoder + vel*Ts;    
    invalid_cnt = invalid_cnt +1;
else
    invalid_cnt = 0;
    encoder_out = encoder;
end

if invalid_cnt>1 
    invalid_cnt = 0;
    encoder_out = encoder;
end

last_valid_encoder = encoder_out;

== matlab function ROPOD_4Wheel_Tdistkinb_cntr_vel_filter_test/Non-ROS Ropod Controller/platform vel cntr/Torque distribution/platform_forces_2_tau_dist_optimal ==
  data: GtSl input; taubody input; ena_w input; Ttaud output; tau_max input; taubody_sc output
function [Ttaud, taubody_sc]   = Ttaud_optimal_vec( GtSl, taubody, ena_w , tau_max)
%#codegen

[Ttaud, taubody_sc]   = tau_optimal_dist_vec_fun( GtSl, taubody, ena_w, tau_max);

end

== matlab function ROPOD_4Wheel_Tdistkinb_cntr_vel_filter_test/Non-ROS Ropod Controller/ROPOD 4SW TORQUE_MODE/ROPOD_4Wheel_sens/Glitch removal + LP filter6/Remove_glitches1 ==
  data: vel input; Ts input; encoder input; encoder_out output
function encoder_out  = remove_glitches(vel, Ts, encoder)

persistent last_valid_encoder;
persistent invalid_cnt;

if(isempty(last_valid_encoder))
    last_valid_encoder = encoder;
    invalid_cnt = 0;
end

if abs( (last_valid_encoder-encoder)/Ts ) > 50 % maximum expected velocity rad/sec (2.5 m/s)
    encoder_out = last_valid_encoder + vel*Ts;    
    invalid_cnt = invalid_cnt +1;
else
    invalid_cnt = 0;
    encoder_out = encoder;
end

if invalid_cnt>1 
    invalid_cnt = 0;
    encoder_out = encoder;
end

last_valid_encoder = encoder_out;

== matlab function ROPOD_4Wheel_Tdistkinb_cntr_vel_filter_test/Non-ROS Ropod Controller/ROPOD 4SW TORQUE_MODE/ROPOD_4Wheel_sens/Glitch removal + LP filter7/Remove_glitches1 ==
  data: vel input; Ts input; encoder input; encoder_out output
function encoder_out  = remove_glitches(vel, Ts, encoder)

persistent last_valid_encoder;
persistent invalid_cnt;

if(isempty(last_valid_encoder))
    last_valid_encoder = encoder;
    invalid_cnt = 0;
end

if abs( (last_valid_encoder-encoder)/Ts ) > 50 % maximum expected velocity rad/sec (2.5 m/s)
    encoder_out = last_valid_encoder + vel*Ts;    
    invalid_cnt = invalid_cnt +1;
else
    invalid_cnt = 0;
    encoder_out = encoder;
end

if invalid_cnt>1 
    invalid_cnt = 0;
    encoder_out = encoder;
end

last_valid_encoder = encoder_out;

== matlab function ROPOD_4Wheel_Tdistkinb_cntr_vel_filter_test/Non-ROS Ropod Controller/ROPOD 4SW TORQUE_MODE/ROPOD_4Wheel_sens/Glitch removal + LP filter9/Remove_glitches1 ==
  data: vel input; Ts input; encoder input; encoder_out output
function encoder_out  = remove_glitches(vel, Ts, encoder)

persistent last_valid_encoder;
persistent invalid_cnt;

if(isempty(last_valid_encoder))
    last_valid_encoder = encoder;
    invalid_cnt = 0;
end

if abs( (last_valid_encoder-encoder)/Ts ) > 50 % maximum expected velocity rad/sec (2.5 m/s)
    encoder_out = last_valid_encoder + vel*Ts;    
    invalid_cnt = invalid_cnt +1;
else
    invalid_cnt = 0;
    encoder_out = encoder;
end

if invalid_cnt>1 
    invalid_cnt = 0;
    encoder_out = encoder;
end

last_valid_encoder = encoder_out;

== matlab function ROPOD_4Wheel_Tdistkinb_cntr_vel_filter_test/Non-ROS Ropod Controller/ROPOD 4SW TORQUE_MODE/ROPOD_4Wheel_sens/Glitch removal + LP filter8/Remove_glitches1 ==
  data: vel input; Ts input; encoder input; encoder_out output
function encoder_out  = remove_glitches(vel, Ts, encoder)

persistent last_valid_encoder;
persistent invalid_cnt;

if(isempty(last_valid_encoder))
    last_valid_encoder = encoder;
    invalid_cnt = 0;
end

if abs( (last_valid_encoder-encoder)/Ts ) > 50 % maximum expected velocity rad/sec (2.5 m/s)
    encoder_out = last_valid_encoder + vel*Ts;    
    invalid_cnt = invalid_cnt +1;
else
    invalid_cnt = 0;
    encoder_out = encoder;
end

if invalid_cnt>1 
    invalid_cnt = 0;
    encoder_out = encoder;
end

last_valid_encoder = encoder_out;

== matlab function ROPOD_4Wheel_Tdistkinb_cntr_vel_filter_test/Non-ROS Ropod Controller/ROPOD 4SW TORQUE_MODE/ROPOD_4Wheel_sens/Glitch removal + LP filter10/Remove_glitches1 ==
  data: vel input; Ts input; encoder input; encoder_out output
function encoder_out  = remove_glitches(vel, Ts, encoder)

persistent last_valid_encoder;
persistent invalid_cnt;

if(isempty(last_valid_encoder))
    last_valid_encoder = encoder;
    invalid_cnt = 0;
end

if abs( (last_valid_encoder-encoder)/Ts ) > 50 % maximum expected velocity rad/sec (2.5 m/s)
    encoder_out = last_valid_encoder + vel*Ts;    
    invalid_cnt = invalid_cnt +1;
else
    invalid_cnt = 0;
    encoder_out = encoder;
end

if invalid_cnt>1 
    invalid_cnt = 0;
    encoder_out = encoder;
end

last_valid_encoder = encoder_out;

== matlab function ROPOD_4Wheel_Tdistkinb_cntr_vel_filter_test/Non-ROS Ropod Controller/ROPOD 4SW TORQUE_MODE/ROPOD_4Wheel_sens/Glitch removal + LP filter11/Remove_glitches1 ==
  data: vel input; Ts input; encoder input; encoder_out output
function encoder_out  = remove_glitches(vel, Ts, encoder)

persistent last_valid_encoder;
persistent invalid_cnt;

if(isempty(last_valid_encoder))
    last_valid_encoder = encoder;
    invalid_cnt = 0;
end

if abs( (last_valid_encoder-encoder)/Ts ) > 50 % maximum expected velocity rad/sec (2.5 m/s)
    encoder_out = last_valid_encoder + vel*Ts;    
    invalid_cnt = invalid_cnt +1;
else
    invalid_cnt = 0;
    encoder_out = encoder;
end

if invalid_cnt>1 
    invalid_cnt = 0;
    encoder_out = encoder;
end

last_valid_encoder = encoder_out;
